simulink model "nucleo_f446_AppShield"  (R2017b)
settings: Solver=FixedStepDiscrete  StartTime=0.0  StopTime=10.0  FixedStep=1e-3  RelTol=1e-3
libraries: mbed_lib x12, simulink x4, mbed_spi_several x1, mbed_i2c_sensors x1
settings Model: Creator=oh  LastModifiedBy=oh
settings DataIOCC: LimitDataPoints=on  SaveFormat=Array
settings OptimizationCC: LifeSpan=1
settings DebuggingCC: SFUnexpectedBacktrackingDiag=warning  SFNoUnconditionalDefaultTransitionDiag=warning  SFExecutionAtInitializationDiag=none
settings HardwareCC: ProdBitPerPointer=32  ProdBitPerSizeT=32  ProdBitPerPtrDiffT=32  ProdLargestAtomicInteger=Long  ProdLargestAtomicFloat=Double  ProdIntDivRoundTo=Undefined  ProdWordSize=32  ProdHWDeviceType=ARM Compatible->ARM Cortex
settings ModelReferenceCC: PropagateSignalLabelsOutOfModel=off
settings SFSimCC: MATLABDynamicMemAlloc=off
settings RTWCC: SystemTargetFile=mbed.tlc  TemplateMakefile=mbed.tmf  Description=Mbed Target (Embedded Target)  TargetLang=C++
settings CodeAppCC: IgnoreCustomStorageClasses=off  StateflowObjectComments=on
settings STFCustomTargetCC: TargetLibSuffix=.a  GenerateSampleERTMain=on  CombineOutputUpdateFcns=on  ERTCustomFileBanners=on  SupportContinuousTime=off  SupportNonInlinedSFcns=off  RemoveResetFunc=on  MATLABClassNameForMDSCustomization=Simulink.SoftwareTarget.ERTCustomization  ModelStepFunctionPrototypeControlCompliant=on  GRTInterface=off  SystemTargetFile=mbed.tlc
settings ERTTargetCC: MultiwordLength=2048  GenerateSampleERTMain=on  ParMdlRefBuildCompliant=off  CompOptLevelCompliant=off  ConcurrentExecutionCompliant=off  CPPClassGenCompliant=off  UseToolchainInfoCompliant=off  ERTCustomFileTemplate=mbed_file_process.tlc  ConvertIfToSwitch=off  SuppressUnreachableDefaultCases=off
settings ConfigComp: CovMetricSettings=dw  CovHtmlReporting=on  CovSaveCumulativeToWorkspaceVar=on  CovSaveSingleToWorkspaceVar=on  CovExternalEMLEnable=off

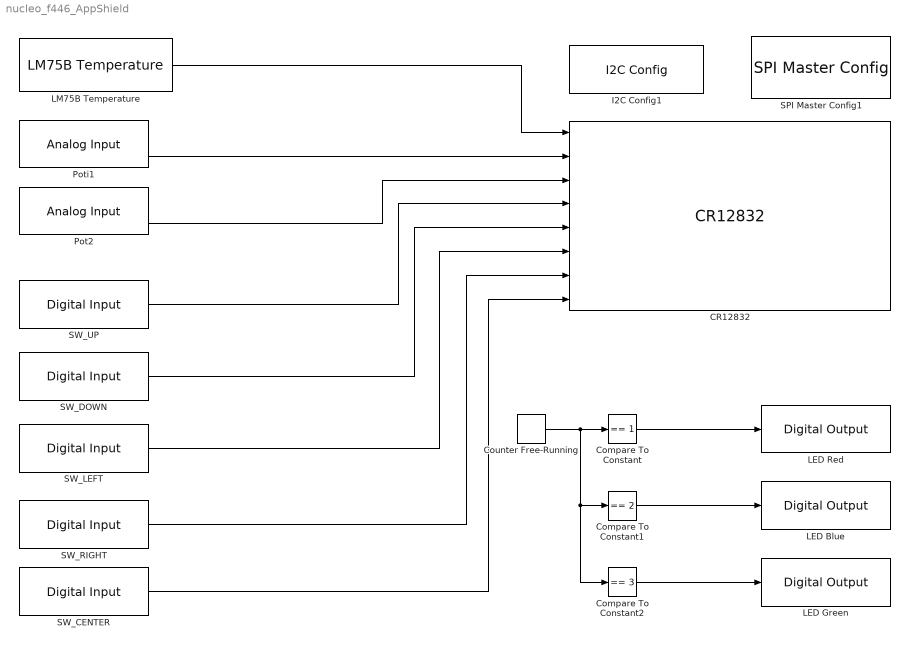
== system nucleo_f446_AppShield ==
  CR12832 : mbed_spi_several/CR12832  TypeOfInputs1={'single'}  NumberOfInputs1=1  Row1='Temperatur %f'  TypeOfInputs2={'single'}  NumberOfInputs2=1  Row2='Poti1 %f'  TypeOfInputs3={'single' 'uint8' 'uint8' 'uint8' 'uint8' 'uint8'}  NumberOfInputs3=6  Row3='Poti2 %f %hu %hu %hu %hu %hu'  SpiPort=1  CsPort=B  CsPin=6  ResPort=A  ResPin=6  A0Port=A  A0Pin=8  SampleTime=0.1
      settings: SourceProductName=Mbed Target
  Compare To Constant : simulink/Logic and Bit Operations/Compare To Constant  relop===  const=1  OutDataTypeStr=uint8
  Compare To Constant1 : simulink/Logic and Bit Operations/Compare To Constant  relop===  const=2  OutDataTypeStr=uint8
  Compare To Constant2 : simulink/Logic and Bit Operations/Compare To Constant  relop===  const=3  OutDataTypeStr=uint8
  Counter Free-Running : simulink/Sources/Counter Free-Running  NumBits=2  tsamp=0.1
  I2C Config1 : mbed_lib/Serial/I2C/I2C Config  Priority=0  I2CPort=1  Freq=100000  SDAPortName=B  SDAPinNumber=9  SCLPortName=B  SCLPinNumber=8
      settings: SourceProductName=Mbed Target
  LED Blue : mbed_lib/GPIO/Digital Output  PortName=A  PinNumber=9  OutputMode=PullDefault  SampleTime=-1
      settings: SourceProductName=Mbed Target
  LED Green : mbed_lib/GPIO/Digital Output  PortName=C  PinNumber=7  OutputMode=PullDefault  SampleTime=-1
      settings: SourceProductName=Mbed Target
  LED Red : mbed_lib/GPIO/Digital Output  PortName=A  PinNumber=10  OutputMode=PullDefault  SampleTime=-1
      settings: SourceProductName=Mbed Target
  LM75B Temperature : mbed_i2c_sensors/LM75B Temperature  I2cPort=1  SampleTime=0.1
      settings: SourceProductName=Mbed Target
  Pot2 : mbed_lib/GPIO/Analog Input  PortName=A  PinNumber=1  SampleTime=0.1
      settings: SourceProductName=Mbed Target
  Poti1 : mbed_lib/GPIO/Analog Input  PortName=A  PinNumber=0  SampleTime=0.1
      settings: SourceProductName=Mbed Target
  SPI Master Config1 : mbed_lib/Serial/SPI/SPI Master Config  Priority=0  SPIPort=1  Freq=100000  Mode=0  Bits=8  MOSIPortNameShow=A  MOSIPortName=0  MOSIPinNumber=7  MISOPortNameShow=A  MISOPortName=0  MISOPinNumber=6  SCLKPortName=A  Parameter13=0  SCLKPinNumber=5
      settings: SourceProductName=Mbed Target
  SW_CENTER : mbed_lib/GPIO/Digital Input  PortName=B  PinNumber=3  InputMode=PullDefault  SampleTime=0.1
      settings: SourceProductName=Mbed Target
  SW_DOWN : mbed_lib/GPIO/Digital Input  PortName=B  PinNumber=0  InputMode=PullDefault  SampleTime=0.1
      settings: SourceProductName=Mbed Target
  SW_LEFT : mbed_lib/GPIO/Digital Input  PortName=C  PinNumber=1  InputMode=PullDefault  SampleTime=0.1
      settings: SourceProductName=Mbed Target
  SW_RIGHT : mbed_lib/GPIO/Digital Input  PortName=C  PinNumber=0  InputMode=PullDefault  SampleTime=0.1
      settings: SourceProductName=Mbed Target
  SW_UP : mbed_lib/GPIO/Digital Input  PortName=A  PinNumber=4  InputMode=PullDefault  SampleTime=0.1
      settings: SourceProductName=Mbed Target
  wires:
  Poti1/2 -> CR12832/2
  Pot2/2 -> CR12832/3
  LM75B Temperature/1 -> CR12832/1
  Counter Free-Running/1 -> Compare To Constant2/1, Compare To Constant1/1, Compare To Constant/1
  Compare To Constant/1 -> LED Red/1
  Compare To Constant1/1 -> LED Blue/1
  Compare To Constant2/1 -> LED Green/1
  SW_UP/1 -> CR12832/4
  SW_DOWN/1 -> CR12832/5
  SW_LEFT/1 -> CR12832/6
  SW_RIGHT/1 -> CR12832/7
  SW_CENTER/1 -> CR12832/8
